simulink model "Lungs_Khoo"  (Simulink 6.4)
settings: Solver=ode45  StartTime=0.0  StopTime=10.0  RelTol=1e-3
values from neighbouring files (symbols this model uses):
  lambda = 863    [Gas_Exchange_IC.m]    (also in Lungs_Khoo_IC.m; Respiratory_IC.m)
  PACO2IC = 37.1484    [Gas_Exchange_IC.m]    (also in Lungs_Khoo_IC.m; Respiratory_IC.m = 40.9432)
  PAO2IC = 107.1983    [Gas_Exchange_IC.m]    (also in Lungs_Khoo_IC.m; Respiratory_IC.m = 102.5153)
  s = 0.000    (= 0)    [Gas_Exchange_IC.m]    (also in Lungs_Khoo_IC.m; Respiratory_IC.m; SaveSimulationSystem.m = fieldnames(x); getPneumonia.m = spline(linspace(0,Simtime,50),rand(1,50)*0.05,t))
  VLCO2 = 3    [Gas_Exchange_IC.m]    (also in Lungs_Khoo_IC.m; Respiratory_IC.m)
  VLO2 = 2.5    [Gas_Exchange_IC.m]    (also in Lungs_Khoo_IC.m; Respiratory_IC.m)
settings Model: LastModifiedBy=CLM
settings OptimizationCC: BlockReduction=off  BooleanDataType=off
settings DebuggingCC: SolverPrmCheckMsg=none  StrictBusMsg=None
settings HardwareCC: TargetUnknown=on

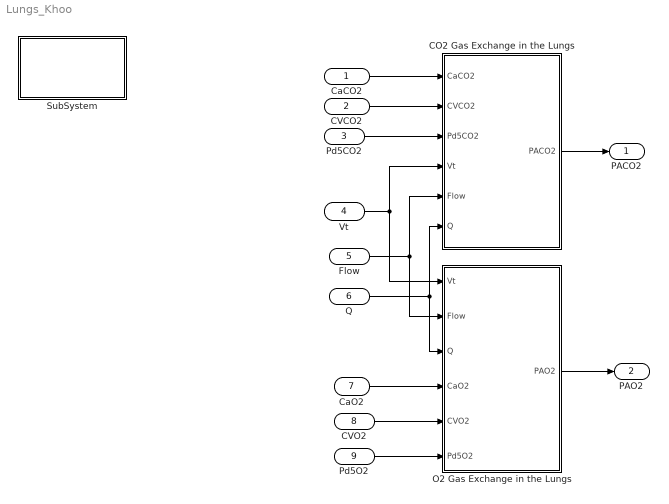
== system Lungs_Khoo ==
  CaCO2 : Inport
  CVCO2 : Inport  Port=2
  Pd5CO2 : Inport  Port=3
  Vt : Inport  Port=4
  Flow : Inport  Port=5
  "Q " : Inport  Port=6
  CaO2 : Inport  Port=7
  CVO2 : Inport  Port=8
  Pd5O2 : Inport  Port=9
  CO2 Gas Exchange in the Lungs : Subsystem
  O2 Gas Exchange in the Lungs : Subsystem
  SubSystem : Subsystem
      settings: OpenFcn=Lungs_Khoo_IC
      mask Display: disp('"double click here"\n to load \nLungs_Khoo \ninitial values');
  PACO2 : Outport
  PAO2 : Outport  Port=2
  wires:
  Pd5O2/1 -> O2 Gas Exchange in the Lungs/6(Pd5O2)
  CVO2/1 -> O2 Gas Exchange in the Lungs/5(CVO2)
  CaO2/1 -> O2 Gas Exchange in the Lungs/4(CaO2)
  "Q "/1 -> CO2 Gas Exchange in the Lungs/6("Q "), O2 Gas Exchange in the Lungs/3("Q ")
  Flow/1 -> CO2 Gas Exchange in the Lungs/5(Flow), O2 Gas Exchange in the Lungs/2(Flow)
  Vt/1 -> CO2 Gas Exchange in the Lungs/4(Vt), O2 Gas Exchange in the Lungs/1(Vt)
  Pd5CO2/1 -> CO2 Gas Exchange in the Lungs/3(Pd5CO2)
  CVCO2/1 -> CO2 Gas Exchange in the Lungs/2(CVCO2)
  CaCO2/1 -> CO2 Gas Exchange in the Lungs/1(CaCO2)
  O2 Gas Exchange in the Lungs/1(PAO2) -> PAO2/1
  CO2 Gas Exchange in the Lungs/1(PACO2) -> PACO2/1

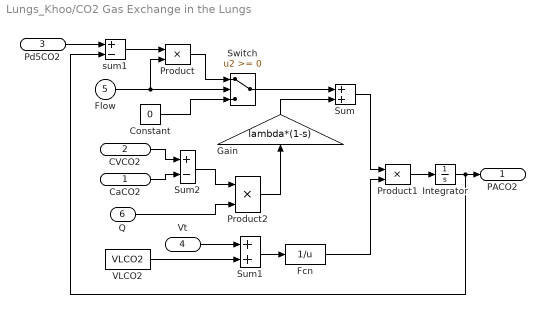
== system Lungs_Khoo/CO2 Gas Exchange in the Lungs ==
  CaCO2 : Inport
  CVCO2 : Inport  Port=2
  Pd5CO2 : Inport  Port=3
  Vt : Inport  Port=4
  Flow : Inport  Port=5
  "Q " : Inport  Port=6
  Constant : Constant  Value=0  OutDataType=sfix(16)  ConRadixGroup=Use specified scaling  OutScaling=2^0  SampleTime=inf  FramePeriod=inf
  Fcn : Fcn  Expr=1/u
  Gain : Gain  Orientation=up  Gain=lambda*(1-s)  SaturateOnIntegerOverflow=on
  Integrator : Integrator  InitialCondition=PACO2IC
  Product : Product  SaturateOnIntegerOverflow=on  RndMeth=Zero  InputSameDT=on
  Product1 : Product  SaturateOnIntegerOverflow=on  RndMeth=Zero  InputSameDT=on
  Product2 : Product  SaturateOnIntegerOverflow=on  RndMeth=Zero  InputSameDT=on
  Sum : Sum  SaturateOnIntegerOverflow=on  InputSameDT=on
  Sum1 : Sum  SaturateOnIntegerOverflow=on  InputSameDT=on
  Sum2 : Sum  Inputs=+-  SaturateOnIntegerOverflow=on  InputSameDT=on
  Switch : Switch  SaturateOnIntegerOverflow=on  InputSameDT=on
  VLCO2 : Constant  Value=VLCO2  OutDataType=sfix(16)  ConRadixGroup=Use specified scaling  OutScaling=2^0  SampleTime=inf  FramePeriod=inf
  sum1 : Sum  Inputs=+-  SaturateOnIntegerOverflow=on  InputSameDT=on
  PACO2 : Outport
  wires:
  Flow/1 -> Product/2, Switch/2
  Vt/1 -> Sum1/1
  Product2/1 -> Gain/1
  "Q "/1 -> Product2/2
  Fcn/1 -> Product1/2
  CVCO2/1 -> Sum2/1
  CaCO2/1 -> Sum2/2
  Sum1/1 -> Fcn/1
  VLCO2/1 -> Sum1/2
  Sum/1 -> Product1/1
  Constant/1 -> Switch/3
  sum1/1 -> Product/1
  Product/1 -> Switch/1
  Switch/1 -> Sum/1
  Product1/1 -> Integrator/1
  Pd5CO2/1 -> sum1/1
  Integrator/1 -> sum1/2, PACO2/1
  Gain/1 -> Sum/2
  Sum2/1 -> Product2/1

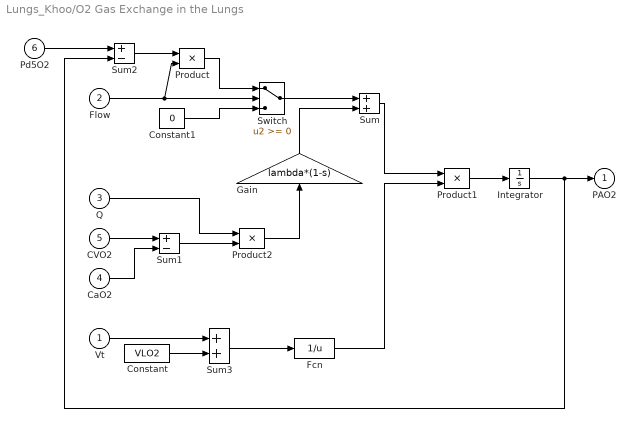
== system Lungs_Khoo/O2 Gas Exchange in the Lungs ==
  Vt : Inport
  Flow : Inport  Port=2
  "Q " : Inport  Port=3
  CaO2 : Inport  Port=4
  CVO2 : Inport  Port=5
  Pd5O2 : Inport  Port=6
  Constant : Constant  Value=VLO2  OutDataType=sfix(16)  ConRadixGroup=Use specified scaling  OutScaling=2^0  SampleTime=inf  FramePeriod=inf
  Constant1 : Constant  Value=0  OutDataType=sfix(16)  ConRadixGroup=Use specified scaling  OutScaling=2^0  SampleTime=inf  FramePeriod=inf
  Fcn : Fcn  Expr=1/u
  Gain : Gain  Orientation=up  Gain=lambda*(1-s)  SaturateOnIntegerOverflow=on
  Integrator : Integrator  InitialCondition=PAO2IC
  Product : Product  SaturateOnIntegerOverflow=on  RndMeth=Zero  InputSameDT=on
  Product1 : Product  SaturateOnIntegerOverflow=on  RndMeth=Zero  InputSameDT=on
  Product2 : Product  SaturateOnIntegerOverflow=on  RndMeth=Zero  InputSameDT=on
  Sum : Sum  SaturateOnIntegerOverflow=on  InputSameDT=on
  Sum1 : Sum  Inputs=+-  SaturateOnIntegerOverflow=on  InputSameDT=on
  Sum2 : Sum  Inputs=+-  SaturateOnIntegerOverflow=on  InputSameDT=on
  Sum3 : Sum  SaturateOnIntegerOverflow=on  InputSameDT=on
  Switch : Switch  SaturateOnIntegerOverflow=on  InputSameDT=on
  PAO2 : Outport
  wires:
  Constant1/1 -> Switch/3
  Product/1 -> Switch/1
  Integrator/1 -> PAO2/1, Sum2/2
  Product1/1 -> Integrator/1
  Constant/1 -> Sum3/2
  Sum3/1 -> Fcn/1
  Fcn/1 -> Product1/2
  Sum2/1 -> Product/1
  Vt/1 -> Sum3/1
  Flow/1 -> Switch/2, Product/2
  CaO2/1 -> Sum1/2
  CVO2/1 -> Sum1/1
  Sum1/1 -> Product2/2
  Product2/1 -> Gain/1
  "Q "/1 -> Product2/1
  Sum/1 -> Product1/1
  Pd5O2/1 -> Sum2/1
  Switch/1 -> Sum/1
  Gain/1 -> Sum/2

== system Lungs_Khoo/SubSystem ==
